simulink model "FIR_FILTER"  (R2018b)
settings: Solver=VariableStepAuto  StartTime=0.0  StopTime=10.0  RelTol=1e-3
libraries: dspsrcs4 x2
settings Model: Creator=MrGoshak  LastModifiedBy=MrGoshak

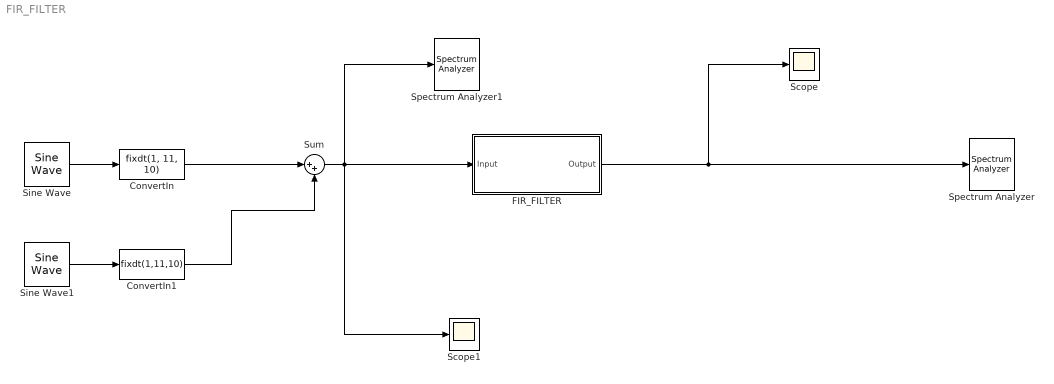
== system FIR_FILTER ==
  ConvertIn : DataTypeConversion  OutDataTypeStr=fixdt(1, 11, 10)  RndMeth=Nearest  SaturateOnIntegerOverflow=on
  ConvertIn1 : DataTypeConversion  OutDataTypeStr=fixdt(1,11,10)  RndMeth=Nearest  SaturateOnIntegerOverflow=on
  FIR_FILTER : Subsystem  Tag=FilterWizardSubSystem
      settings: ErrorFcn=dspFilterRealizedInBasicElemsAlgLoopErrFcnCallback
  Scope : Scope
  Scope1 : Scope
  Sine Wave : dspsrcs4/Sine Wave  Amplitude=1/2  Frequency=10000  Phase=0  SampleMode=Discrete  OutComplex=Real  CompMethod=Trigonometric fcn  TableSize=Speed  SampleTime=1/500000  SamplesPerFrame=1  ResetState=Restart at time zero  OutputFrames=off  dataType=double  wordLen=16  udDataType=sfix(16)  fracBitsMode=Best precision  numFracBits=15  OutDataTypeStr=double  LastOutDataTypeStr=double
  Sine Wave1 : dspsrcs4/Sine Wave  Amplitude=1/2  Frequency=60000  Phase=0  SampleMode=Discrete  OutComplex=Real  CompMethod=Trigonometric fcn  TableSize=Speed  SampleTime=1/500000  SamplesPerFrame=1  ResetState=Restart at time zero  OutputFrames=off  dataType=double  wordLen=16  udDataType=sfix(16)  fracBitsMode=Best precision  numFracBits=15  OutDataTypeStr=double  LastOutDataTypeStr=double
  Spectrum Analyzer : SpectrumAnalyzer
  Spectrum Analyzer1 : SpectrumAnalyzer
  Sum : Sum  Inputs=|++  OutDataTypeStr=fixdt(1,12,11)  SaturateOnIntegerOverflow=on  InputSameDT=on
  wires:
  FIR_FILTER/1(Output) -> Scope/1, Spectrum Analyzer/1
  Sum/1 -> Spectrum Analyzer1/1, FIR_FILTER/1(Input), Scope1/1
  Sine Wave/1 -> ConvertIn/1
  Sine Wave1/1 -> ConvertIn1/1
  ConvertIn/1 -> Sum/1
  ConvertIn1/1 -> Sum/2

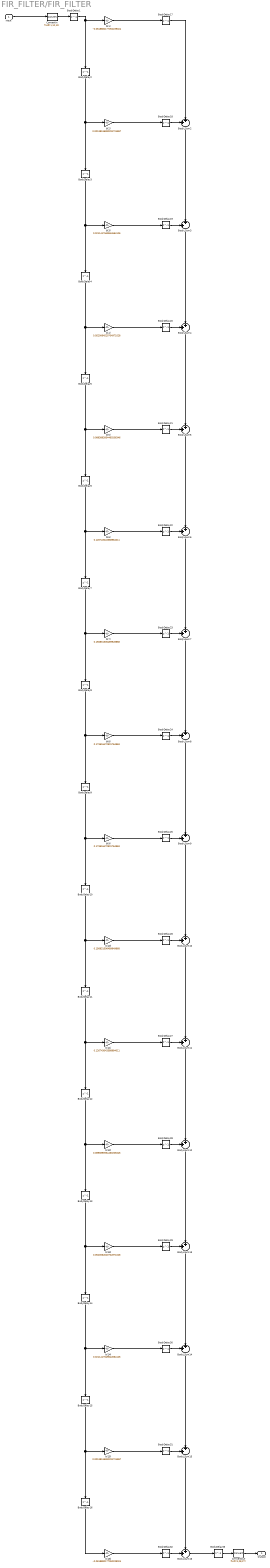
== system FIR_FILTER/FIR_FILTER ==
  Input : Inport
  BodyDelay{1..33} (33 alike) : Delay  DelayLength=1  InitialCondition=0
  BodyLSum{2..16} (15 alike) : Sum  Inputs=++|  AccumDataTypeStr=fixdt(1,28,26)  OutDataTypeStr=fixdt(1,28,27)  SaturateOnIntegerOverflow=on
  ConvertIn : DataTypeConversion  OutDataTypeStr=fixdt(1,12,11)  RndMeth=Nearest  SaturateOnIntegerOverflow=on
  ConvertOut : DataTypeConversion  OutDataTypeStr=fixdt(1,28,27)  SaturateOnIntegerOverflow=on
  b(1) : Gain  Gain=-0.0618882177052239024  ParamDataTypeStr=fixdt(1,16,15)  OutDataTypeStr=fixdt(1,28,27)  SaturateOnIntegerOverflow=on
  b(10) : Gain  Gain=0.156831506489949868  ParamDataTypeStr=fixdt(1,16,15)  OutDataTypeStr=fixdt(1,28,27)  SaturateOnIntegerOverflow=on
  b(11) : Gain  Gain=0.126743043388984011  ParamDataTypeStr=fixdt(1,16,15)  OutDataTypeStr=fixdt(1,28,27)  SaturateOnIntegerOverflow=on
  b(12) : Gain  Gain=0.0893893934460206346  ParamDataTypeStr=fixdt(1,16,15)  OutDataTypeStr=fixdt(1,28,27)  SaturateOnIntegerOverflow=on
  b(13) : Gain  Gain=0.0520064520704971028  ParamDataTypeStr=fixdt(1,16,15)  OutDataTypeStr=fixdt(1,28,27)  SaturateOnIntegerOverflow=on
  b(14) : Gain  Gain=0.0211417649844564126  ParamDataTypeStr=fixdt(1,16,15)  OutDataTypeStr=fixdt(1,28,27)  SaturateOnIntegerOverflow=on
  b(15) : Gain  Gain=0.00138246382291724867  ParamDataTypeStr=fixdt(1,16,15)  OutDataTypeStr=fixdt(1,28,27)  SaturateOnIntegerOverflow=on
  b(16) : Gain  Gain=-0.0618882177052239024  ParamDataTypeStr=fixdt(1,16,15)  OutDataTypeStr=fixdt(1,28,27)  SaturateOnIntegerOverflow=on
  b(2) : Gain  Gain=0.00138246382291724867  ParamDataTypeStr=fixdt(1,16,15)  OutDataTypeStr=fixdt(1,28,27)  SaturateOnIntegerOverflow=on
  b(3) : Gain  Gain=0.0211417649844564126  ParamDataTypeStr=fixdt(1,16,15)  OutDataTypeStr=fixdt(1,28,27)  SaturateOnIntegerOverflow=on
  b(4) : Gain  Gain=0.0520064520704971028  ParamDataTypeStr=fixdt(1,16,15)  OutDataTypeStr=fixdt(1,28,27)  SaturateOnIntegerOverflow=on
  b(5) : Gain  Gain=0.0893893934460206346  ParamDataTypeStr=fixdt(1,16,15)  OutDataTypeStr=fixdt(1,28,27)  SaturateOnIntegerOverflow=on
  b(6) : Gain  Gain=0.126743043388984011  ParamDataTypeStr=fixdt(1,16,15)  OutDataTypeStr=fixdt(1,28,27)  SaturateOnIntegerOverflow=on
  b(7) : Gain  Gain=0.156831506489949868  ParamDataTypeStr=fixdt(1,16,15)  OutDataTypeStr=fixdt(1,28,27)  SaturateOnIntegerOverflow=on
  b(8) : Gain  Gain=0.173616470901764963  ParamDataTypeStr=fixdt(1,16,15)  OutDataTypeStr=fixdt(1,28,27)  SaturateOnIntegerOverflow=on
  b(9) : Gain  Gain=0.173616470901764963  ParamDataTypeStr=fixdt(1,16,15)  OutDataTypeStr=fixdt(1,28,27)  SaturateOnIntegerOverflow=on
  Output : Outport
  wires:
  Input/1 -> ConvertIn/1
  b(1)/1 -> BodyDelay17/1
  ConvertIn/1 -> BodyDelay1/1
  BodyDelay2/1 -> b(2)/1, BodyDelay3/1
  b(2)/1 -> BodyDelay18/1
  BodyLSum2/1 -> BodyLSum3/2
  BodyDelay3/1 -> b(3)/1, BodyDelay4/1
  b(3)/1 -> BodyDelay19/1
  BodyLSum3/1 -> BodyLSum4/2
  BodyDelay4/1 -> b(4)/1, BodyDelay5/1
  b(4)/1 -> BodyDelay20/1
  BodyLSum4/1 -> BodyLSum5/2
  BodyDelay5/1 -> b(5)/1, BodyDelay6/1
  b(5)/1 -> BodyDelay21/1
  BodyLSum5/1 -> BodyLSum6/2
  BodyDelay6/1 -> b(6)/1, BodyDelay7/1
  b(6)/1 -> BodyDelay22/1
  BodyLSum6/1 -> BodyLSum7/2
  BodyDelay7/1 -> b(7)/1, BodyDelay8/1
  b(7)/1 -> BodyDelay23/1
  BodyLSum7/1 -> BodyLSum8/2
  BodyDelay8/1 -> b(8)/1, BodyDelay9/1
  b(8)/1 -> BodyDelay24/1
  BodyLSum8/1 -> BodyLSum9/2
  BodyDelay9/1 -> b(9)/1, BodyDelay10/1
  b(9)/1 -> BodyDelay25/1
  BodyLSum9/1 -> BodyLSum10/2
  BodyDelay10/1 -> b(10)/1, BodyDelay11/1
  b(10)/1 -> BodyDelay26/1
  BodyLSum10/1 -> BodyLSum11/2
  BodyDelay11/1 -> b(11)/1, BodyDelay12/1
  b(11)/1 -> BodyDelay27/1
  BodyLSum11/1 -> BodyLSum12/2
  BodyDelay12/1 -> b(12)/1, BodyDelay13/1
  b(12)/1 -> BodyDelay28/1
  BodyLSum12/1 -> BodyLSum13/2
  BodyDelay13/1 -> b(13)/1, BodyDelay14/1
  b(13)/1 -> BodyDelay29/1
  BodyLSum13/1 -> BodyLSum14/2
  BodyDelay14/1 -> b(14)/1, BodyDelay15/1
  b(14)/1 -> BodyDelay30/1
  BodyLSum14/1 -> BodyLSum15/2
  BodyDelay15/1 -> b(15)/1, BodyDelay16/1
  b(15)/1 -> BodyDelay31/1
  BodyLSum15/1 -> BodyLSum16/1
  BodyDelay16/1 -> b(16)/1
  b(16)/1 -> BodyDelay32/1
  ConvertOut/1 -> Output/1
  BodyDelay1/1 -> b(1)/1, BodyDelay2/1
  BodyDelay17/1 -> BodyLSum2/2
  BodyDelay18/1 -> BodyLSum2/1
  BodyDelay19/1 -> BodyLSum3/1
  BodyDelay20/1 -> BodyLSum4/1
  BodyDelay21/1 -> BodyLSum5/1
  BodyDelay22/1 -> BodyLSum6/1
  BodyDelay23/1 -> BodyLSum7/1
  BodyDelay24/1 -> BodyLSum8/1
  BodyDelay25/1 -> BodyLSum9/1
  BodyDelay26/1 -> BodyLSum10/1
  BodyDelay27/1 -> BodyLSum11/1
  BodyDelay28/1 -> BodyLSum12/1
  BodyDelay29/1 -> BodyLSum13/1
  BodyDelay30/1 -> BodyLSum14/1
  BodyDelay31/1 -> BodyLSum15/1
  BodyDelay32/1 -> BodyLSum16/2
  BodyLSum16/1 -> BodyDelay33/1
  BodyDelay33/1 -> ConvertOut/1
